simulink model "Filling_Model"  (R2022b)
settings: Solver=FixedStepAuto  StartTime=0.0  StopTime=inf  FixedStep=0.02  RelTol=1e-3
undefined symbols (not defined in the file or in its folder): amount, B, KePhi, Ra, tau_a, tau_m
libraries: slpidlib x1
settings Model: Creator=omar  LastModifiedBy=omar

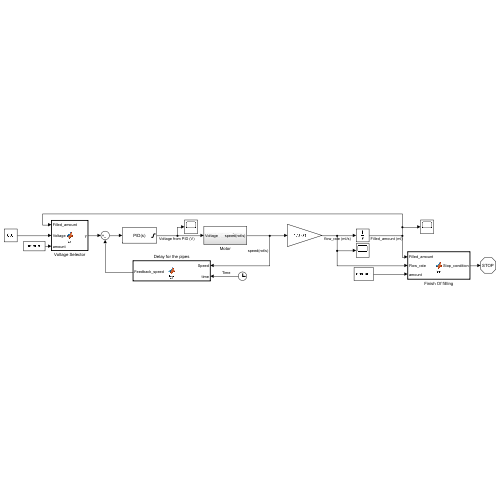
[thumbnail: Simulink's stored preview of the top-level diagram]
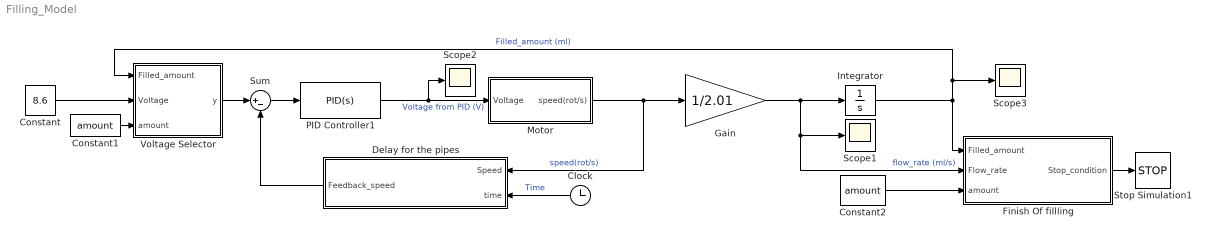
== system Filling_Model ==
  Clock : Clock
  Constant : Constant  Value=8.6
  Constant1 : Constant  Value=amount
  Constant2 : Constant  Value=amount
  Delay for the pipes : MATLAB Function  TreatAsAtomicUnit=on
  Finish Of fillling : MATLAB Function  TreatAsAtomicUnit=on
  Gain : Gain  Gain=1/2.01
  Integrator : Integrator
  Motor : Subsystem
  PID Controller1 : slpidlib/PID Controller  Controller=PID  Form=Parallel  TimeDomain=Continuous-time  UseExternalTs=off  SampleTime=-1  IntegratorMethod=Forward Euler  FilterMethod=Forward Euler  ControllerParametersSource=internal  P=12  I=12  UseKiTs=off  D=0.1  N=100  UseFilter=on  TunerSelectOption=Transfer Function Based (PID Tuner App)  InitialConditionSource=internal  InitialConditionForIntegrator=0  InitialConditionForFilter=0  DifferentiatorICPrevScaledInput=0  ExternalReset=none  TrackingMode=off  Kt=1  LimitOutput=on  SatLimitsSource=internal  UpperSaturationLimit=10  LowerSaturationLimit=0  LinearizeAsGain=on  AntiWindupMode=none  Kb=1  LimitIntegrator=off  UpperIntegratorSaturationLimit=inf  LowerIntegratorSaturationLimit=-inf  POutMin=[]  POutMax=[]  IOutMin=[]  IOutMax=[]  DOutMin=[]  DOutMax=[]  NOutMin=[]  NOutMax=[]  SumOutMin=[]  SumOutMax=[]  SaturationOutMin=[]  SaturationOutMax=[]  PParamMin=[]  PParamMax=[]  IParamMin=[]  IParamMax=[]  DParamMin=[]  DParamMax=[]  NParamMin=[]  NParamMax=[]  KbParamMin=[]  KbParamMax=[]  KtParamMin=[]  KtParamMax=[]  KbOutMin=[]  KbOutMax=[]  KtOutMin=[]  KtOutMax=[]  IntegratorOutMin=[]  IntegratorOutMax=[]  FilterOutMin=[]  FilterOutMax=[]  SumI1OutMin=[]  SumI1OutMax=[]  SumI2OutMin=[]  SumI2OutMax=[]  SumI3OutMin=[]  SumI3OutMax=[]  SumI4OutMin=[]  SumI4OutMax=[]  SumDOutMin=[]  SumDOutMax=[]  DifferentiatorOutMin=[]  DifferentiatorOutMax=[]  FilterDiffOutCoefMin=[]  FilterDiffOutCoefMax=[]  ReciprocalOutMin=[]  ReciprocalOutMax=[]  SumDenOutMin=[]  SumDenOutMax=[]  SumNumOutMin=[]  SumNumOutMax=[]  DivideOutMin=[]  DivideOutMax=[]  UdiffTsProdOutMin=[]  UdiffTsProdOutMax=[]  NTsProdOutMin=[]  NTsProdOutMax=[]  UintegralTsProdOutMin=[]  UintegralTsProdOutMax=[]  UngainTsProdOutMin=[]  UngainTsProdOutMax=[]  ClampingZeroOutDataTypeStr=Inherit: Inherit via back propagation  ClampingZeroOutMin=[]  ClampingZeroOutMax=[]  FilterDenConstantOutDataTypeStr=Inherit: Inherit via back propagation  FilterDenConstantOutMin=[]  FilterDenConstantOutMax=[]  PCopyOutDataTypeStr=Inherit: Inherit via back propagation  PCopyOutMin=[]  PCopyOutMax=[]  NCopyOutDataTypeStr=Inherit: Inherit via back propagation  NCopyOutMin=[]  NCopyOutMax=[]  IntegratorContinuousStateAttributes=''  IntegratorStateMustResolveToSignalObject=off  IntegratorRTWStateStorageClass=Auto  FilterContinuousStateAttributes=''  FilterStateMustResolveToSignalObject=off  FilterRTWStateStorageClass=Auto  ParallelPVariant=InternalParameters  IdealPVariant=Disabled  IVariant=InternalParameters  DVariant=InternalParameters  IntegratorVariant=Continuous  SatVariant=Enabled  AWVariant=Passthrough  PCopyVariant=Disabled  TRVariant=Disabled  FdbkBlocksVariant=Forward  IdealPFdbkVariant=Disabled  SatFdbkVariant=Disabled  DerivativeFilterVariant=ContFilter  NVariant=InternalParameters  NCopyVariant=Disabled  FilterICVariant=InternalICsFilter  IntegratorICVariant=InternalICs  ExternalResetVariant=Disabled  TRSumVariant=Passthrough  SumFdbkVariant=Disabled  SumVariant=Sum_PID  TsampFilterVariant=InternalTs  TsampNgainVariant=Passthrough  TsampIntegralVariant=Passthrough  ExternalSaturationOutDataTypeStr=Inherit: Same as second input
  Scope1 : Scope
  Scope2 : Scope
  Scope3 : Scope
  Stop Simulation1 : Stop
  Sum : Sum  Inputs=|+-
  Voltage Selector : MATLAB Function  TreatAsAtomicUnit=on
  wires:
  Delay for the pipes/1(Feedback_speed) -> Sum/2
  PID Controller1/1 -> Scope2/1, Motor/1(Voltage)  "Voltage from PID (V)"
  Integrator/1 -> Scope3/1, Voltage Selector/1(Filled_amount), Finish Of fillling/1(Filled_amount)  "Filled_amount (ml)"
  Constant/1 -> Voltage Selector/2(Voltage)
  Constant1/1 -> Voltage Selector/3(amount)
  Constant2/1 -> Finish Of fillling/3(amount)
  Finish Of fillling/1(Stop_condition) -> Stop Simulation1/1
  Gain/1 -> Integrator/1, Scope1/1, Finish Of fillling/2(Flow_rate)  "flow_rate (ml/s)"
  Sum/1 -> PID Controller1/1
  Motor/1(speed(rot/s)) -> Delay for the pipes/1(Speed), Gain/1  "speed(rot/s)"
  Clock/1 -> Delay for the pipes/2(time)  "Time"
  Voltage Selector/1(y) -> Sum/1

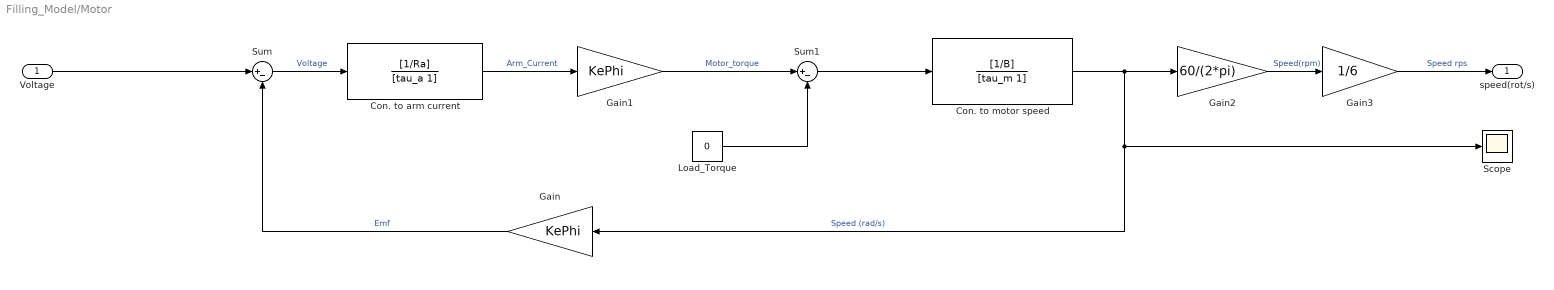
== system Filling_Model/Motor ==
  Voltage : Inport  OutMin=[0]  OutMax=[10]
  Con. to arm current : TransferFcn  Numerator=[1/Ra]  Denominator=[tau_a 1]
  Con. to motor speed : TransferFcn  Numerator=[1/B]  Denominator=[tau_m 1]
  Gain : Gain  Gain=KePhi
  Gain1 : Gain  Gain=KePhi
  Gain2 : Gain  Gain=60/(2*pi)
  Gain3 : Gain  Gain=1/6
  Load_Torque : Constant  Value=0
  Scope : Scope
  Sum : Sum  Inputs=|+-
  Sum1 : Sum  Inputs=|+-
  speed(rot/s) : Outport
  wires:
  Gain1/1 -> Sum1/1  "Motor_torque"
  Sum/1 -> Con. to arm current/1  "Voltage"
  Load_Torque/1 -> Sum1/2
  Gain2/1 -> Gain3/1  "Speed(rpm)"
  Gain/1 -> Sum/2  "Emf"
  Con. to arm current/1 -> Gain1/1  "Arm_Current"
  Gain3/1 -> speed(rot/s)/1  "Speed rps"
  Con. to motor speed/1 -> Scope/1, Gain/1, Gain2/1  "Speed (rad/s)"
  Sum1/1 -> Con. to motor speed/1
  Voltage/1 -> Sum/1

== matlab function Filling_Model/Delay for the pipes ==
  data: Speed input; Feedback_speed output; time input
function Feedback_speed = fcn(Speed,time)
if(time<2)
Speed = 0 ;  
end
Feedback_speed = Speed;

== matlab function Filling_Model/Voltage Selector ==
  data: Filled_amount input; Voltage input; y output; amount input
function y = fcn( Filled_amount,Voltage, amount)
if(amount <=30)
    factor = 0.79;
elseif(amount<=35)
    factor = 0.84;
elseif(amount<=40)
    factor = 0.88;
elseif(amount<=45)
    factor = 0.89;
elseif(amount<=50)
    factor = 0.9;
elseif(amount<=75)
    factor = 0.93;
elseif(amount<=100)
    factor = 0.96;
elseif(amount<=125)
    factor = 0.97;    
else
    factor = 0.98;
end
if(Filled_amount>= amount*factor)
    Voltage = 0 ; 
end
y = Voltage;

== matlab function Filling_Model/Finish Of fillling ==
  data: Filled_amount input; Flow_rate input; Stop_condition output; amount input
function Stop_condition = fcn(Filled_amount, Flow_rate, amount)
t=0;
if((Flow_rate<=0.01) &&(Filled_amount>=amount*0.98))
   t=1;
end

Stop_condition = t;
